simulink model "EV_FlexibleShaft"  (R2026a)
settings: Solver=ode45  StopTime=FlexibleStopTime  MaxStep=FlexibleMaxStep  RelTol=FlexibleRelTol  AbsTol=FlexibleAbsTol
values from neighbouring files (symbols this model uses):
  Ip = 1    [RigidShaft_parameters.m]
  k = 10    [RigidShaft_parameters.m]
  Ks = G*Jpolar/shaft_length    [FlexibleShaft_parameters.m]
  L = 1    [RigidShaft_parameters.m]
  L_effective = L + k^2/Ks    [FlexibleShaft_parameters.m]
  R = 1    [RigidShaft_parameters.m]
  t_step_M = 0.8    [RigidShaft_parameters.m]
  t_step_V = 0.1    [RigidShaft_parameters.m]
settings Model: Creator=dinul  LastModifiedBy=dinul

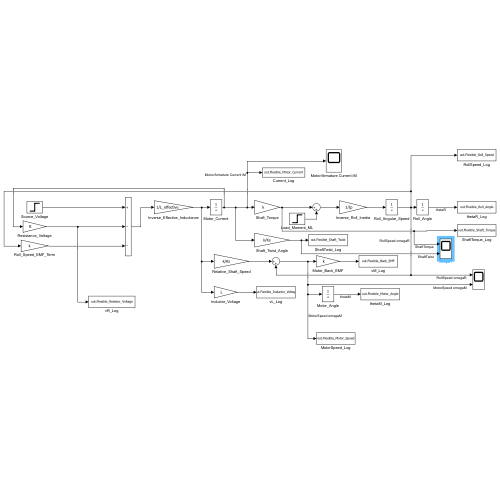
[thumbnail: Simulink's stored preview of the top-level diagram]
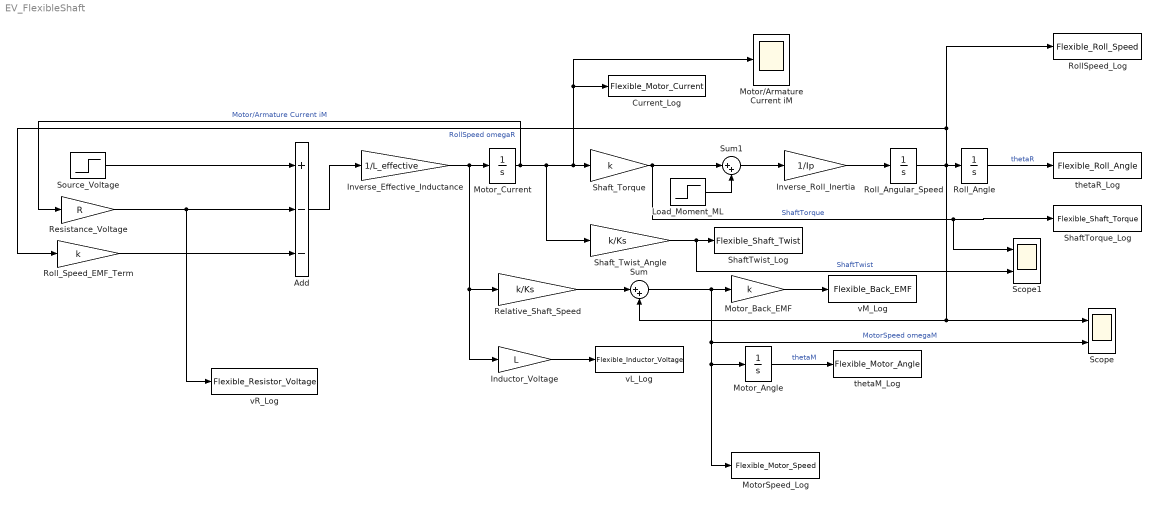
== system EV_FlexibleShaft ==
  Add : Sum  Inputs=+--
  Current_Log : ToWorkspace  VariableName=Flexible_Motor_Current  SaveFormat=Timeseries  SampleTime=-1
  Inductor_Voltage : Gain  Gain=L
  Inverse_Effective_Inductance : Gain  Gain=1/L_effective
  Inverse_Roll_Inertia : Gain  Gain=1/Ip
  Load_Moment_ML : Step  Time=t_step_M  FinalValue=ML_flexible_model_amp  SampleTime=0
  Motor/Armature Current iM : Scope
      settings: ActiveDisplayYMinimum=-0.094045376608300119  ActiveDisplayYMaximum=0.10555041852531623
  MotorSpeed_Log : ToWorkspace  VariableName=Flexible_Motor_Speed  SaveFormat=Timeseries  SampleTime=-1
  Motor_Angle : Integrator
  Motor_Back_EMF : Gain  Gain=k
  Motor_Current : Integrator
  Relative_Shaft_Speed : Gain  Gain=k/Ks
  Resistance_Voltage : Gain  Gain=R
  RollSpeed_Log : ToWorkspace  VariableName=Flexible_Roll_Speed  SaveFormat=Timeseries  SampleTime=-1
  Roll_Angle : Integrator
  Roll_Angular_Speed : Integrator
  Roll_Speed_EMF_Term : Gain  Gain=k
  Scope : Scope  NumInputPorts=2
      settings: ActiveDisplayYMinimum=-0.023319652482450902  ActiveDisplayYMaximum=0.20987687234205815
  Scope1 : Scope  NumInputPorts=2
      settings: ActiveDisplayYMinimum=-0.94045376608300135  ActiveDisplayYMaximum=1.0555041852531621  DataLoggingVariableName=ScopeData2
  ShaftTorque_Log : ToWorkspace  VariableName=Flexible_Shaft_Torque  SaveFormat=Timeseries  SampleTime=-1
  ShaftTwist_Log : ToWorkspace  VariableName=Flexible_Shaft_Twist  SaveFormat=Timeseries  SampleTime=-1
  Shaft_Torque : Gain  Gain=k
  Shaft_Twist_Angle : Gain  Gain=k/Ks
  Source_Voltage : Step  Time=t_step_V  FinalValue=Vs_step_amp  SampleTime=0
  Sum : Sum  Inputs=|++
  Sum1 : Sum  Inputs=|++
  thetaM_Log : ToWorkspace  VariableName=Flexible_Motor_Angle  SaveFormat=Timeseries  SampleTime=-1
  thetaR_Log : ToWorkspace  VariableName=Flexible_Roll_Angle  SaveFormat=Timeseries  SampleTime=-1
  vL_Log : ToWorkspace  VariableName=Flexible_Inductor_Voltage  SaveFormat=Timeseries  SampleTime=-1
  vM_Log : ToWorkspace  VariableName=Flexible_Back_EMF  SaveFormat=Timeseries  SampleTime=-1
  vR_Log : ToWorkspace  VariableName=Flexible_Resistor_Voltage  SaveFormat=Timeseries  SampleTime=-1
  wires:
  Source_Voltage/1 -> Add/1
  Add/1 -> Inverse_Effective_Inductance/1
  Inverse_Effective_Inductance/1 -> Inductor_Voltage/1, Relative_Shaft_Speed/1, Motor_Current/1
  Motor_Current/1 -> Motor/Armature Current iM/1, Current_Log/1, Shaft_Torque/1, Shaft_Twist_Angle/1, Resistance_Voltage/1  "Motor/Armature Current iM"
  Resistance_Voltage/1 -> vR_Log/1, Add/2
  Roll_Angular_Speed/1 -> Roll_Speed_EMF_Term/1, RollSpeed_Log/1, Sum/2, Scope/1, Roll_Angle/1  "RollSpeed omegaR"
  Roll_Speed_EMF_Term/1 -> Add/3
  Shaft_Torque/1 -> Sum1/1, ShaftTorque_Log/1, Scope1/1  "ShaftTorque"
  Load_Moment_ML/1 -> Sum1/2
  Sum1/1 -> Inverse_Roll_Inertia/1
  Inverse_Roll_Inertia/1 -> Roll_Angular_Speed/1
  Relative_Shaft_Speed/1 -> Sum/1
  Sum/1 -> MotorSpeed_Log/1, Motor_Angle/1, Scope/2, Motor_Back_EMF/1  "MotorSpeed omegaM"
  Shaft_Twist_Angle/1 -> Scope1/2, ShaftTwist_Log/1  "ShaftTwist"
  Inductor_Voltage/1 -> vL_Log/1
  Motor_Back_EMF/1 -> vM_Log/1
  Roll_Angle/1 -> thetaR_Log/1  "thetaR"
  Motor_Angle/1 -> thetaM_Log/1  "thetaM"
